simulink model "c"  (R2012b)
settings: Solver=ode45  StartTime=0.0  StopTime=100  RelTol=1e-3
settings Model: Creator=ZhouHaoyu  LastModifiedBy=ZhouHaoyu

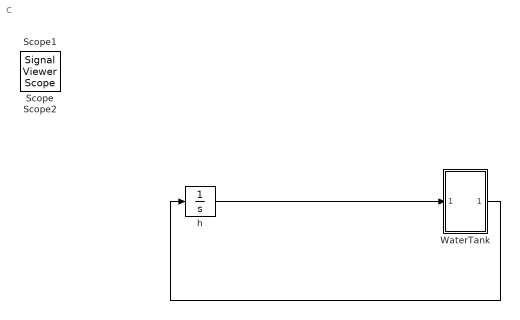
== system c ==
  WaterTank : Subsystem
  h : Integrator  LimitOutput=on  UpperSaturationLimit=2  LowerSaturationLimit=0
  Scope : SignalViewerScope  IOType=viewer  RefreshTime=0.035000
  Scope1 : SignalViewerScope  IOType=viewer  RefreshTime=0.035000
  Scope2 : SignalViewerScope  IOType=viewer  RefreshTime=0.035000
      settings: SaveName=ScopeData2
  wires:
  h/1 -> WaterTank/1(In1)
  WaterTank/1(Out1) -> h/1

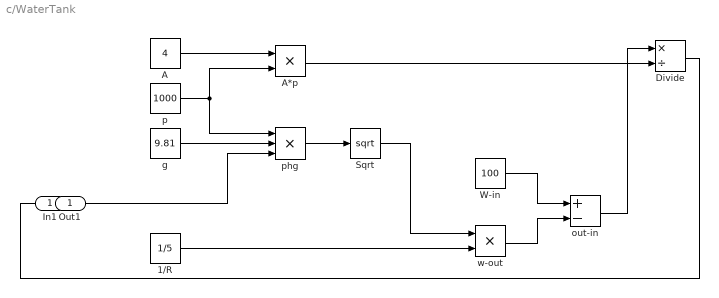
== system c/WaterTank ==
  In1 : Inport
  1/R : Constant  Value=1/5
  A : Constant  Value=4
  A*p : Product  RndMeth=Zero
  Divide : Product  Inputs=*/
  Sqrt : Sqrt  SaturateOnIntegerOverflow=on
  W-in : Constant  Value=100
  g : Constant  Value=9.81
  out-in : Sum  Inputs=+-
  p : Constant  Value=1000
  "phg " : Product  Inputs=3  RndMeth=Zero
  w-out : Product  RndMeth=Zero
  Out1 : Outport
  wires:
  A/1 -> A*p/1
  p/1 -> A*p/2, "phg "/1
  g/1 -> "phg "/2
  "phg "/1 -> Sqrt/1
  Sqrt/1 -> w-out/1
  1/R/1 -> w-out/2
  In1/1 -> "phg "/3
  W-in/1 -> out-in/1
  w-out/1 -> out-in/2
  out-in/1 -> Divide/1
  A*p/1 -> Divide/2
  Divide/1 -> Out1/1
